simulink model "control2"  (R2021a)
settings: Solver=VariableStepAuto  StartTime=0.0  StopTime=10  RelTol=1e-3
undefined symbols (not defined in the file): D
libraries: simulink x1
settings Model: Creator=caios  LastModifiedBy=caios

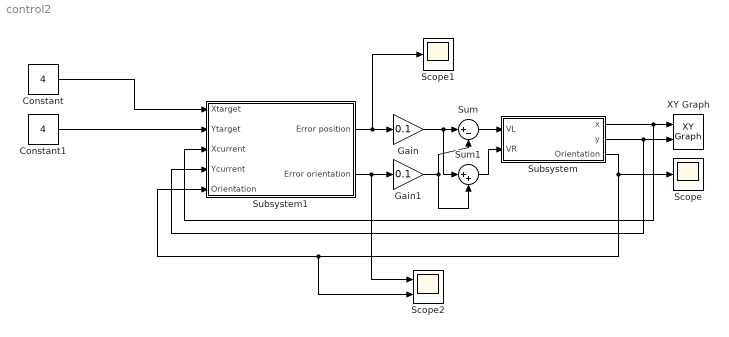
== system control2 ==
  Constant : Constant  Value=4
  Constant1 : Constant  Value=4
  Gain : Gain  Gain=0.1
  Gain1 : Gain  Gain=0.1
  Scope : Scope
  Scope1 : Scope
  Scope2 : Scope  NumInputPorts=2
  Subsystem : Subsystem
  Subsystem1 : Subsystem
  Sum : Sum  Inputs=|+-
  Sum1 : Sum  Inputs=|++
  XY Graph : simulink/Sinks/XY Graph  xmin=-10  xmax=10  ymin=-10  ymax=10  st=-1
  wires:
  Subsystem/3(Orientation) -> Scope2/2, Subsystem1/5(Orientation), Scope/1
  Subsystem/1(x) -> Subsystem1/3(Xcurrent), XY Graph/1
  Subsystem/2(y) -> Subsystem1/4(Ycurrent), XY Graph/2
  Constant/1 -> Subsystem1/1(Xtarget)
  Constant1/1 -> Subsystem1/2(Ytarget)
  Subsystem1/1(Error position) -> Scope1/1, Gain/1
  Gain/1 -> Sum1/1, Sum/1
  Sum/1 -> Subsystem/1(VL)
  Subsystem1/2(Error orientation) -> Scope2/1, Gain1/1
  Gain1/1 -> Sum1/2, Sum/2
  Sum1/1 -> Subsystem/2(VR)

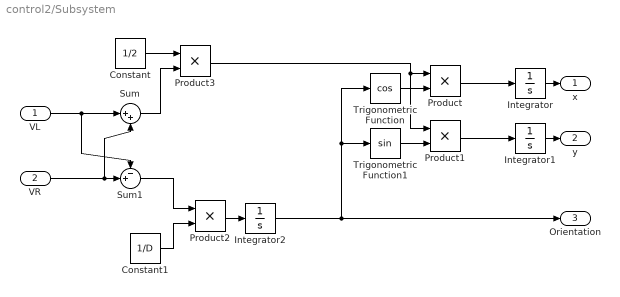
== system control2/Subsystem ==
  VL : Inport
  VR : Inport  Port=2
  Constant : Constant  Value=1/2
  Constant1 : Constant  Value=1/D
  Integrator : Integrator
  Integrator1 : Integrator
  Integrator2 : Integrator
  Product{,1..3} (4 alike) : Product
  Sum : Sum  Inputs=|++
  Sum1 : Sum  Inputs=-+|
  Trigonometric Function : Trigonometry  Operator=cos
  Trigonometric Function1 : Trigonometry
  x : Outport
  y : Outport  Port=2
  Orientation : Outport  Port=3
  wires:
  Integrator/1 -> x/1
  Integrator1/1 -> y/1
  Integrator2/1 -> Trigonometric Function/1, Trigonometric Function1/1, Orientation/1
  Product2/1 -> Integrator2/1
  Constant1/1 -> Product2/2
  Sum1/1 -> Product2/1
  Constant/1 -> Product3/1
  Sum/1 -> Product3/2
  VL/1 -> Sum/1, Sum1/1
  VR/1 -> Sum1/2, Sum/2
  Trigonometric Function/1 -> Product/2
  Trigonometric Function1/1 -> Product1/2
  Product1/1 -> Integrator1/1
  Product3/1 -> Product1/1, Product/1
  Product/1 -> Integrator/1

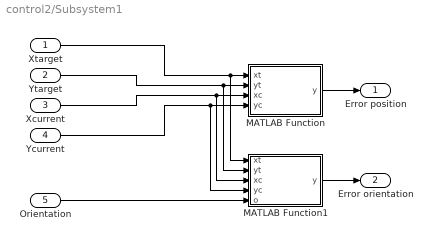
== system control2/Subsystem1 ==
  Xtarget : Inport
  Ytarget : Inport  Port=2
  Xcurrent : Inport  Port=3
  Ycurrent : Inport  Port=4
  Orientation : Inport  Port=5
  MATLAB Function : MATLAB Function  TreatAsAtomicUnit=on
  MATLAB Function1 : MATLAB Function  TreatAsAtomicUnit=on
  Error position : Outport
  Error orientation : Outport  Port=2
  wires:
  Xtarget/1 -> MATLAB Function1/1(xt), MATLAB Function/1(xt)
  Ytarget/1 -> MATLAB Function1/2(yt), MATLAB Function/2(yt)
  Xcurrent/1 -> MATLAB Function1/3(xc), MATLAB Function/3(xc)
  Ycurrent/1 -> MATLAB Function1/4(yc), MATLAB Function/4(yc)
  MATLAB Function/1(y) -> Error position/1
  Orientation/1 -> MATLAB Function1/5(o)
  MATLAB Function1/1(y) -> Error orientation/1

== matlab function control2/Subsystem1/MATLAB Function1 ==
  data: xt input; y output; yt input; xc input; yc input; o input
function y = fcn(xt,yt,xc,yc,o)
dy = yt-yc;
dx = xt-xc;
theta = atan(dy/dx);
y=theta-o;

== matlab function control2/Subsystem1/MATLAB Function ==
  data: xt input; y output; yt input; xc input; yc input
function y = fcn(xt,yt,xc,yc)

y = sqrt((xt-xc)^2+(yt-yc)^2);
